simulink model "PubIfDecisionTOS_MDL"  (R2020b)
settings: configuration reference "DspaceConfig" (kept outside this file)
PostLoadFcn:
  | if any(exist('dsrtsu_mdlpostloadfcn', 'file') ~= 0), dsrtsu_mdlpostloadfcn('Execute', bdroot); end
InitFcn:
  | , if any(exist('dsmpb_private', 'file') ~= 0), dsmpb_private('dsmpb_mdlclblib', 'Init', bdroot); end,
undefined symbols (not defined in the file or in its folder): C_TOS_ACCEgoRAxletoFbumplength_m, C_TOS_ACCTargetFront_Flag, C_TOS_AEBJAPedObjDxThre_Val, C_TOS_AEBJAPedObjDyThre_Val, C_TOS_AEBJATargetSize_Val, C_TOS_AEBJAVehObjDxThre_Val, C_TOS_AEBJAVehObjDyThre_Val, C_TOS_AEBJuncPedTargetSize_Val, C_TOS_AEBLatObjDxThre_Val, C_TOS_AEBLatPedDyThre_Val, C_TOS_AEBLatTargetSize_Val, C_TOS_AEBLongTargetInEgoFront_Flag, C_TOS_axAbsGround_Parameter, C_TOS_CameraConfirmedFlag, C_TOS_CNsubjWidth, C_TOS_CurrentLaneCoreMinWidth_Val, C_TOS_CutInProb_Val_Zero, C_TOS_CutOutProb_Val_Zero, C_TOS_D2R_Val, C_TOS_DefaultValueObjectToCenterLine_dy, C_TOS_EgoCarWidth_Val, C_TOS_EgoDxRefPoint_m, C_TOS_EgoRAxletoFbumplength_m, C_TOS_HalfWidthVehicle_Con, C_TOS_HWA_CurrentLaneFlag, C_TOS_HWA_LeftLaneFlag, C_TOS_HWA_MovingDir_Vaild, C_TOS_HWA_MovState_Vaild, C_TOS_HWA_RightLaneFlag, C_TOS_LaneLineCourseErrorFront, C_TOS_LaneLineCourseErrorRear, C_TOS_MotorbikeDefaultWidth_m, C_TOS_NumberOfEffectiveTargets, C_TOS_Obj_Age_Val, C_TOS_Objdx_Constraint_Val, C_TOS_ObjectDefaultWidth_m, C_TOS_ObjInCurrentLane_Val, C_TOS_ObjInCurrentLaneValid, C_TOS_ObjInLeftLaneValid, C_TOS_ObjInRightLaneValid, C_TOS_ObjNotInCurrentLane_Val, C_TOS_ObjNotREElementType, C_TOS_ObjPredictDis_dy_ConstantVal_Zeros, C_TOS_ObjToCenterLine_ConstantVal_Zeros, C_TOS_OFMObjIDInvilad_Val, C_TOS_PIL_LatDisCons_Val_zero, C_TOS_PIL_ObjectCutInFlag_b, C_TOS_PIL_ObjectCutOutFlag_b, C_TOS_PIL_ObjLaneProb_al_Val, C_TOS_PP_ObjFusType_FC_Confirm_b, C_TOS_PP_ObjFusType_FC_FR_Confirm_b, C_TOS_PP_ObjFusType_FR_Confirm_b, C_TOS_RE_80BoolDefault_Val, C_TOS_RE_80Single181Default_Val, C_TOS_RE_80Single255Default_Val, C_TOS_RE_80Uint8Default_Val, C_TOS_RE_D2R, C_TOS_RE_D_180_Val, C_TOS_RE_InvalidObjectID_Val, C_TOS_RE_InvalidTargetChainDir_Val ... (+142)
libraries: simulink x1650, TOS_LIB x361, canfdmsglib x14
(part 11 of 69)

== system PubIfDecisionTOS_MDL/TOS_20201112/TOS_2012080320/PP1128/ISV_InputSignalVerification/LM_SignalVerif/LM_RR_Bus ==
  LM_LINE_RR : Inport
  Bus Creator2 : BusCreator  Inputs=8  OutDataTypeStr=Bus: TOS_LM_RR_Line_bus  NonVirtualBus=on
      settings: InheritFromInputs=off
  Bus Selector1 : BusSelector  OutputSignals=LM_Line01,LM_Line02,LM_Line03,LM_Line04,LM_Line05,LM_Line06,LM_Line07,LM_Line08
  LM_RR_Line01 : Subsystem
  LM_RR_Line02 : Subsystem
  LM_RR_Line03 : Subsystem
  LM_RR_Line04 : Subsystem
  LM_RR_Line05 : Subsystem
  LM_RR_Line06 : Subsystem
  LM_RR_Line07 : Subsystem
  LM_RR_Line08 : Subsystem
  LM_RR_Bus : Outport
  wires:
  LM_LINE_RR/1 -> Bus Selector1/1
  LM_RR_Line03/1(LM_RR_Line03) -> Bus Creator2/3  "LM_RR_Line03"
  LM_RR_Line02/1(LM_RR_Line02) -> Bus Creator2/2  "LM_RR_Line02"
  Bus Selector1/8 -> LM_RR_Line08/1(LM_Line08)  "<LM_Line08>"
  LM_RR_Line06/1(LM_RR_Line06) -> Bus Creator2/6  "LM_RR_Line06"
  LM_RR_Line04/1(LM_RR_Line04) -> Bus Creator2/4  "LM_RR_Line04"
  LM_RR_Line08/1(LM_RR_Line08) -> Bus Creator2/8  "LM_RR_Line08"
  Bus Selector1/2 -> LM_RR_Line02/1(LM_Line02)  "<LM_Line02>"
  Bus Selector1/6 -> LM_RR_Line06/1(LM_Line06)  "<LM_Line06>"
  LM_RR_Line05/1(LM_RR_Line05) -> Bus Creator2/5  "LM_RR_Line05"
  Bus Selector1/3 -> LM_RR_Line03/1(LM_Line03)  "<LM_Line03>"
  Bus Selector1/7 -> LM_RR_Line07/1(LM_Line07)  "<LM_Line07>"
  Bus Creator2/1 -> LM_RR_Bus/1
  LM_RR_Line01/1(LM_RR_Line01) -> Bus Creator2/1  "LM_RR_Line01"
  Bus Selector1/4 -> LM_RR_Line04/1(LM_Line04)  "<LM_Line04>"
  Bus Selector1/5 -> LM_RR_Line05/1(LM_Line05)  "<LM_Line05>"
  Bus Selector1/1 -> LM_RR_Line01/1(LM_Line01)  "<LM_Line01>"
  LM_RR_Line07/1(LM_RR_Line07) -> Bus Creator2/7  "LM_RR_Line07"

== system PubIfDecisionTOS_MDL/TOS_20201112/TOS_2012080320/TLJ/Pro/Pro/ObjInLane ==
  Object_Type : Inport
  Object_DY : Inport  Port=2
  PIL_CutinFlag : Inport  Port=3
  PIL_CutoutFlag : Inport  Port=4
  "PIL_EgoVehicleInLeftlaneProb  " : Inport  Port=5
  "PIL_EgoVehicleInMiddlelaneProb  " : Inport  Port=6
  "PIL_EgoVehicleInRightlaneProb  " : Inport  Port=7
  "PIL_ObjinLeftLaneProb " : Inport  Port=8
  PIL_ObjinEgoLaneProb : Inport  Port=9
  "PIL_ObjInRightlaneProb " : Inport  Port=10
  "TLJ_ObjinLeftLaneProb " : Inport  Port=11
  TLJ_ObjinEgoLaneProb : Inport  Port=12
  "TLJ_ObjInRightlaneProb " : Inport  Port=13
  Bus Creator1 : BusCreator  Inputs=13
  Bus Selector : BusSelector  OutputSignals=ObjInLeftLane_flag,ObjInEgoLane_flag,ObjInRightLane_flag,TOS_TLJ_ObjInLaneCondition_Flag_ObserVale
  Bus Selector1 : BusSelector  OutputSignals=Object_Type,TLJ_ObjinEgoLaneProb,TLJ_ObjinLeftLaneProb,TLJ_ObjInRightlaneProb,PIL_CutinFlag,PIL_CutoutFlag,Object_DY
  Bus Selector2 : BusSelector  OutputSignals=TLJ_ObjinEgoLaneProb,TLJ_ObjinLeftLaneProb,TLJ_ObjInRightlaneProb
  Bus Selector3 : BusSelector  OutputSignals=TLJ_ObjinEgoLaneProb,TLJ_ObjinLeftLaneProb,TLJ_ObjInRightlaneProb
  Bus Selector4 : BusSelector  OutputSignals=PIL_ObjinEgoLaneProb,PIL_ObjinLeftLaneProb,PIL_EgoVehicleInLeftlaneProb,PIL_EgoVehicleInMiddlelaneProb
  Bus Selector5 : BusSelector  OutputSignals=PIL_ObjinEgoLaneProb,PIL_ObjInRightlaneProb,PIL_EgoVehicleInRightlaneProb,PIL_EgoVehicleInMiddlelaneProb
  ObjInEgoLane_flag_1 : Subsystem  TreatAsAtomicUnit=on
  ObjInEgoLane_flag_2 : Subsystem  TreatAsAtomicUnit=on
  ObjInEgoLane_flag_3 : Subsystem  TreatAsAtomicUnit=on
  ObjInLane_Default : Subsystem  TreatAsAtomicUnit=on
  ObjInLeftLane_flag : Subsystem  TreatAsAtomicUnit=on
  ObjInRightLane_flag : Subsystem  TreatAsAtomicUnit=on
  Switch{,1..4} (5 alike) : Switch  Criteria=u2 > Threshold
  TLJ_ObjInEgoLane_1 : Subsystem
  TLJ_ObjInEgoLane_2 : Subsystem
  TLJ_ObjInEgoLane_3 : Subsystem
  TLJ_ObjInLeftLane : Subsystem
  TLJ_ObjInRightLane : Subsystem
  TLJ_ObjInLeftLane_flag : Outport
  TLJ_ObjInEgoLane_flag : Outport  Port=2
  TLJ_ObjInRightLane_flag : Outport  Port=3
  TOS_TLJ_ObjInLaneCondition_Flag_ObserVale : Outport  Port=4
  wires:
  ObjInLane_Default/1(ObjInEgoLane_flag_2) -> Switch4/3
  ObjInEgoLane_flag_1/1(ObjInEgoLane_flag_1) -> Switch/1
  Bus Selector5/3 -> TLJ_ObjInEgoLane_3/3("PIL_EgoVehicleInRightlaneProb  ")  "<PIL_EgoVehicleInRightlaneProb>"
  TLJ_ObjInEgoLane_3/1(TLJ_ObjInRightLane_flag) -> Switch4/2  "TLJ_ObjInEgoLane_3"
  Bus Selector2/1 -> TLJ_ObjInLeftLane/1(TLJ_ObjinEgoLaneProb)  "<TLJ_ObjinEgoLaneProb>"
  "PIL_EgoVehicleInLeftlaneProb  "/1 -> Bus Creator1/5  "PIL_EgoVehicleInLeftlaneProb"
  Bus Selector3/2 -> TLJ_ObjInRightLane/2(TLJ_ObjinLeftLaneProb)  "<TLJ_ObjinLeftLaneProb>"
  PIL_CutinFlag/1 -> Bus Creator1/3  "PIL_CutinFlag"
  Bus Selector3/3 -> TLJ_ObjInRightLane/3(TLJ_ObjinRightLaneProb)  "<TLJ_ObjInRightlaneProb>"
  Switch4/1 -> Switch3/3
  TLJ_ObjInLeftLane/1(TLJ_ObjInLeftLane_flag) -> Switch1/2  "TLJ_ObjInLeftLane"
  Switch/1 -> Bus Selector/1
  TLJ_ObjInEgoLane_2/1(TLJ_ObjInRightLane_flag) -> Switch3/2  "TLJ_ObjInEgoLane_2"
  TLJ_ObjInRightLane/1(TLJ_ObjInRightLane_flag) -> Switch2/2  "TLJ_ObjInRightLane"
  ObjInEgoLane_flag_3/1(ObjInEgoLane_flag_1) -> Switch4/1
  TLJ_ObjInEgoLane_1/1(TLJ_ObjInEgoLane_flag) -> Switch/2  "TLJ_ObjInEgoLane_1"
  ObjInRightLane_flag/1(ObjInRightLane_flag) -> Switch2/1
  Bus Selector1/4 -> TLJ_ObjInEgoLane_1/4("TLJ_ObjInRightlaneProb ")  "<TLJ_ObjInRightlaneProb>"
  ObjInEgoLane_flag_2/1(ObjInEgoLane_flag_1) -> Switch3/1
  Bus Selector5/1 -> TLJ_ObjInEgoLane_3/1("PIL_ObjinEgoLaneProb ")  "<PIL_ObjinEgoLaneProb>"
  Bus Creator1/1 -> Bus Selector5/1, Bus Selector4/1, Bus Selector3/1, Bus Selector2/1, Bus Selector1/1
  Bus Selector1/1 -> TLJ_ObjInEgoLane_1/1(Object_Type)  "<Object_Type>"
  Object_Type/1 -> Bus Creator1/1  "Object_Type"
  "PIL_EgoVehicleInMiddlelaneProb  "/1 -> Bus Creator1/6  "PIL_EgoVehicleInMiddlelaneProb"
  TLJ_ObjinEgoLaneProb/1 -> Bus Creator1/12  "TLJ_ObjinEgoLaneProb"
  Bus Selector4/3 -> TLJ_ObjInEgoLane_2/3("PIL_EgoVehicleInLeftlaneProb  ")  "<PIL_EgoVehicleInLeftlaneProb>"
  "PIL_EgoVehicleInRightlaneProb  "/1 -> Bus Creator1/7  "PIL_EgoVehicleInRightlaneProb"
  Bus Selector1/5 -> TLJ_ObjInEgoLane_1/5(PIL_CutinFlag)  "<PIL_CutinFlag>"
  "TLJ_ObjInRightlaneProb "/1 -> Bus Creator1/13  "TLJ_ObjInRightlaneProb"
  Bus Selector2/3 -> TLJ_ObjInLeftLane/3(TLJ_ObjinRightLaneProb)  "<TLJ_ObjInRightlaneProb>"
  "TLJ_ObjinLeftLaneProb "/1 -> Bus Creator1/11  "TLJ_ObjinLeftLaneProb"
  Bus Selector4/1 -> TLJ_ObjInEgoLane_2/1("PIL_ObjinEgoLaneProb ")  "<PIL_ObjinEgoLaneProb>"
  Switch3/1 -> Switch2/3
  Bus Selector2/2 -> TLJ_ObjInLeftLane/2("TLJ_ObjinLeftLaneProb ")  "<TLJ_ObjinLeftLaneProb>"
  ObjInLeftLane_flag/1(ObjInLeftLane_flag) -> Switch1/1
  Bus Selector3/1 -> TLJ_ObjInRightLane/1(TLJ_ObjinEgoLaneProb)  "<TLJ_ObjinEgoLaneProb>"
  Bus Selector4/4 -> TLJ_ObjInEgoLane_2/4("PIL_EgoVehicleInMiddlelaneProb  ")  "<PIL_EgoVehicleInMiddlelaneProb>"
  Switch1/1 -> Switch/3
  Bus Selector4/2 -> TLJ_ObjInEgoLane_2/2("PIL_ObjInLeftlaneProb ")  "<PIL_ObjinLeftLaneProb>"
  Switch2/1 -> Switch1/3
  Bus Selector1/2 -> TLJ_ObjInEgoLane_1/2(TLJ_ObjinEgoLaneProb)  "<TLJ_ObjinEgoLaneProb>"
  Bus Selector5/2 -> TLJ_ObjInEgoLane_3/2("PIL_ObjInRightlaneProb ")  "<PIL_ObjInRightlaneProb>"
  Bus Selector1/3 -> TLJ_ObjInEgoLane_1/3("TLJ_ObjinLeftLaneProb ")  "<TLJ_ObjinLeftLaneProb>"
  Bus Selector5/4 -> TLJ_ObjInEgoLane_3/4("PIL_EgoVehicleInMiddlelaneProb  ")  "<PIL_EgoVehicleInMiddlelaneProb>"
  Bus Selector/1 -> TLJ_ObjInLeftLane_flag/1  "<ObjInLeftLane_flag>"
  Bus Selector/2 -> TLJ_ObjInEgoLane_flag/1  "<ObjInEgoLane_flag>"
  Bus Selector/3 -> TLJ_ObjInRightLane_flag/1  "<ObjInRightLane_flag>"
  "PIL_ObjinLeftLaneProb "/1 -> Bus Creator1/8  "PIL_ObjinLeftLaneProb"
  PIL_ObjinEgoLaneProb/1 -> Bus Creator1/9  "PIL_ObjinEgoLaneProb"
  "PIL_ObjInRightlaneProb "/1 -> Bus Creator1/10  "PIL_ObjInRightlaneProb"
  Bus Selector/4 -> TOS_TLJ_ObjInLaneCondition_Flag_ObserVale/1  "<TOS_TLJ_ObjInLaneCondition_Flag_ObserVale>"
  Object_DY/1 -> Bus Creator1/2  "Object_DY"
  Bus Selector1/7 -> TLJ_ObjInEgoLane_1/7(Object_DY)  "<Object_DY>"
  PIL_CutoutFlag/1 -> Bus Creator1/4  "PIL_CutoutFlag"
  Bus Selector1/6 -> TLJ_ObjInEgoLane_1/6(PIL_CutoutFlag)  "<PIL_CutoutFlag>"

== system PubIfDecisionTOS_MDL/TOS_20201112/TOS_2012080320/TLJ/Pro/Pro/Pro ==
  PIL_EgoLaneProb : Inport
  PIL_LeftLaneProb : Inport  Port=2
  PIL_RightLaneProb : Inport  Port=3
  PIL_EgoVehicle_EgoLaneProb : Inport  Port=4
  PIL_EgoVehicle_LeftLaneProb : Inport  Port=5
  PIL_EgoVehicle_RightLaneProb : Inport  Port=6
  Add1 : Sum  OutDataTypeStr=single
  Add2 : Sum  OutDataTypeStr=single
  Add3 : Sum  Inputs=+++  OutDataTypeStr=single
  Bus Creator : BusCreator  Inputs=6
  Bus Selector : BusSelector  OutputSignals=ObjLaneProb_ix_i0,EgoLaneProb_i0,ObjLaneProb_ix_i1,EgoLaneProb_i1,ObjLaneProb_ix_i2,EgoLaneProb_i2
  Bus Selector1 : BusSelector  OutputSignals=ObjLaneProb_ix_i0,EgoLaneProb_i1,ObjLaneProb_ix_i1,EgoLaneProb_i2
  Bus Selector2 : BusSelector  OutputSignals=ObjLaneProb_ix_i1,EgoLaneProb_i0,ObjLaneProb_ix_i2,EgoLaneProb_i1
  Product{1..7} (7 alike) : Product
  TLJ_ObjinLeftLaneProb : Outport
  TLJ_ObjinEgoLaneProb : Outport  Port=2
  TLJ_ObjinRightLaneProb : Outport  Port=3
  wires:
  Add1/1 -> TLJ_ObjinLeftLaneProb/1
  Bus Selector1/2 -> Product3/2  "<EgoLaneProb_i1>"
  Bus Selector/1 -> Product1/1  "<ObjLaneProb_ix_i0>"
  Bus Selector1/3 -> Product4/1  "<ObjLaneProb_ix_i1>"
  PIL_LeftLaneProb/1 -> Bus Creator/1  "ObjLaneProb_ix_i0"
  Bus Selector/6 -> Product7/2  "<EgoLaneProb_i2>"
  Bus Selector/2 -> Product1/2  "<EgoLaneProb_i0>"
  Product7/1 -> Add3/3
  Product1/1 -> Add3/1
  Bus Selector1/1 -> Product3/1  "<ObjLaneProb_ix_i0>"
  PIL_EgoVehicle_EgoLaneProb/1 -> Bus Creator/5  "EgoLaneProb_i1"
  Bus Selector/5 -> Product7/1  "<ObjLaneProb_ix_i2>"
  Bus Creator/1 -> Bus Selector2/1, Bus Selector1/1, Bus Selector/1
  PIL_EgoVehicle_RightLaneProb/1 -> Bus Creator/6  "EgoLaneProb_i2"
  Bus Selector/4 -> Product2/2  "<EgoLaneProb_i1>"
  Add3/1 -> TLJ_ObjinEgoLaneProb/1
  PIL_EgoVehicle_LeftLaneProb/1 -> Bus Creator/4  "EgoLaneProb_i0"
  Product6/1 -> Add2/2
  Bus Selector/3 -> Product2/1  "<ObjLaneProb_ix_i1>"
  PIL_RightLaneProb/1 -> Bus Creator/3  "ObjLaneProb_ix_i2"
  Bus Selector2/1 -> Product5/1  "<ObjLaneProb_ix_i1>"
  Product4/1 -> Add1/2
  Product2/1 -> Add3/2
  Bus Selector1/4 -> Product4/2  "<EgoLaneProb_i2>"
  PIL_EgoLaneProb/1 -> Bus Creator/2  "ObjLaneProb_ix_i1"
  Bus Selector2/3 -> Product6/1  "<ObjLaneProb_ix_i2>"
  Product3/1 -> Add1/1
  Product5/1 -> Add2/1
  Bus Selector2/2 -> Product5/2  "<EgoLaneProb_i0>"
  Add2/1 -> TLJ_ObjinRightLaneProb/1
  Bus Selector2/4 -> Product6/2  "<EgoLaneProb_i1>"

== system PubIfDecisionTOS_MDL/TOS_20201112/TOS_2012080320/TOS/ACC/TOS_ACCCurrentLane/ACCTargetInfor ==
  note: TOS_ProbInLaneCalculat 信号未使用
  OFM_SignalVerification : Inport
  TOS_AddAttributes : Inport  Port=2
  TOS_ProbInLaneCalculat : Inport  Port=3
  TOS_ACCP0TargetIndex : Inport  Port=4  OutDataTypeStr=uint8
  TOS_ACCP1TargetIndex : Inport  Port=5  OutDataTypeStr=uint8
  Bus Creator : BusCreator  Inputs=3
  Bus Selector : BusSelector  OutputSignals=OFM_SignalVerification,TOS_AddAttributes,TOS_ProbInLaneCalculat
  Bus Selector1 : BusSelector  OutputSignals=OFM_SignalVerification,TOS_AddAttributes
  Bus Selector2 : BusSelector  OutputSignals=IDP0
  TOS_ACCP0TargetInfor : Stateflow chart  TreatAsAtomicUnit=on
  TOS_ACCP1TargetInfor : Stateflow chart  TreatAsAtomicUnit=on
  TOS_ACCP0 : Outport  PortDimensions=1  BusOutputAsStruct=on
  TOS_ACCP1 : Outport  Port=2
  wires:
  TOS_ACCP1TargetInfor/1(TOS_ACCPO1TargetInfo) -> TOS_ACCP1/1
  Bus Selector1/2 -> TOS_ACCP1TargetInfor/3(TOS_AddAttributes)  "<TOS_AddAttributes>"
  Bus Selector1/1 -> TOS_ACCP1TargetInfor/2(OFM_SignalVerification)  "<OFM_SignalVerification>"
  TOS_ACCP0TargetInfor/1(TOS_ACCPO0TargetInfo) -> Bus Selector2/1, TOS_ACCP0/1
  Bus Selector/3 -> TOS_ACCP0TargetInfor/3(TOS_ProbInLaneCalculat)  "<TOS_ProbInLaneCalculat>"
  TOS_ProbInLaneCalculat/1 -> Bus Creator/3  "TOS_ProbInLaneCalculat"
  OFM_SignalVerification/1 -> Bus Creator/1  "OFM_SignalVerification"
  TOS_AddAttributes/1 -> Bus Creator/2  "TOS_AddAttributes"
  Bus Selector/2 -> TOS_ACCP0TargetInfor/2(TOS_AddAttributes)  "<TOS_AddAttributes>"
  Bus Selector/1 -> TOS_ACCP0TargetInfor/1(OFM_SignalVerification)  "<OFM_SignalVerification>"
  Bus Selector2/1 -> [TOS_ACCP0_ID]  "<IDP0>"
  TOS_ACCP0TargetIndex/1 -> TOS_ACCP0TargetInfor/4(TOS_ACCPO0TargetIndex)
  TOS_ACCP1TargetIndex/1 -> TOS_ACCP1TargetInfor/4(TOS_ACCPO1TargetIndex)
  [TOS_ACCP0_ID] -> TOS_ACCP1TargetInfor/1(IDP0)
  Bus Creator/1 -> Bus Selector1/1, Bus Selector/1

== system PubIfDecisionTOS_MDL/TOS_20201112/TOS_2012080320/TOS/ACC/TOS_ACCCurrentLane/ACC_CurrentLane_Target ==
  VIE_EgoVelocity : Inport
  OFM_SignalVerification : Inport  Port=2
  TOS_AddAttributes : Inport  Port=3
  TOS_TLJ_SameLaneConfirm_Flag : Inport  Port=4
  TOS_ProbInLaneCalculat : Inport  Port=5
  TOS_VCAN_SignalVerification : Inport  Port=6
  LM_LR_Line04_dDisStart : Inport  Port=7
  LM_LR_Line04_dDisEnd : Inport  Port=8
  LM_LR_Line05_dDisStart : Inport  Port=9
  LM_LR_Line05_dDisEnd : Inport  Port=10
  LM_LR_Line06_dDisStart : Inport  Port=11
  LM_LR_Line06_dDisEnd : Inport  Port=12
  LM_LR_Line04_pC2 : Inport  Port=13
  LM_LR_Line05_pC2 : Inport  Port=14
  LM_LR_Line06_pC2 : Inport  Port=15
  LM_LR_Line04_fCamValid : Inport  Port=16
  LM_LR_Line05_fCamValid : Inport  Port=17
  LM_LR_Line06_fCamValid : Inport  Port=18
  LM_LR_Line04_pC0 : Inport  Port=19
  LM_RL_Line04_pC0 : Inport  Port=20
  LM_LR_Line04_pC1 : Inport  Port=21
  LM_RL_Line04_pC1 : Inport  Port=22
  ACC_P0_P1_Index : Inport  Port=23
  ACC_TargetP0_ID_K1 : Inport  Port=24
  ACC_TargetP0_MovState_K1 : Inport  Port=25
  ACC_TargetP1_ID_K1 : Inport  Port=26
  ACC_TargetP1_MovState_K1 : Inport  Port=27
  ACC_TargetP0_ID_K2 : InportShadow  Port=24
  ACC_TargetP0_MovState_K2 : InportShadow  Port=25
  ACC_TargetP1_ID_K2 : InportShadow  Port=26
  ACC_TargetP1_MovState_K2 : InportShadow  Port=27
  Bus Creator : BusCreator  Inputs=31
  Bus Creator1 : BusCreator  Inputs=18
  Bus Creator2 : BusCreator  Inputs=18
  Bus Selector : BusSelector  OutputSignals=ACC_P0_P1_Index,OFM_SignalVerification.Object_ID,OFM_SignalVerification.Object_Fus_Type,OFM_SignalVerification.Object_MovingState,TOS_AddAttributes.PP_ObjMovingDirSignalProcessing,OFM_SignalVerification.Object_HeadingAngle,OFM_SignalVerification.Object_DX,TOS_TLJ_SameLaneConfirm_Flag,OFM_SignalVerification.Object_Type,OFM_SignalVerification.Object_ObstacleProb,OFM_SignalVerification.Object_DY,TOS_AddAttributes.PP_ObjFusType_FC_FR_Confirm,TOS_AddAttributes.PP_ObjFusType_FR_Confirm,TOS_AddAttributes.PP_ObjFusType_FC_Confirm,OFM_SignalVerification.Object_VX,OFM_SignalVerification.Object_VY,VIE_EgoVelocity,TOS_VCAN_SignalVerification.SteerWheelAng,TOS_ProbInLaneCalculat.PIL_OverlapRatio,ACC_TargetP0_ID_K1,ACC_TargetP0_ID_K2,ACC_TargetP0_MovState_K1,ACC_TargetP0_MovState_K2,LM_LR_Line04_dDisStart,LM_LR_Line04_dDisEnd,LM_LR_Line05_dDisStart,LM_LR_Line05_dDisEnd,LM_LR_Line06_dDisStart,LM_LR_Line06_dDisEnd,LM_LR_Line04_pC2,LM_LR_Line05_pC2,LM_LR_Line06_pC2,LM_LR_Line04_fCamValid,LM_LR_Line05_fCamValid,LM_LR_Line06_fCamValid,LM_LR_Line04_pC0,LM_RL_Line04_pC0,LM_LR_Line04_pC1,LM_RL_Line04_pC1
  Bus Selector2 : BusSelector  OutputSignals=ACC_P0_P1_Index,OFM_SignalVerification.Object_ID,OFM_SignalVerification.Object_Fus_Type,OFM_SignalVerification.Object_MovingState,TOS_AddAttributes.PP_ObjMovingDirSignalProcessing,OFM_SignalVerification.Object_HeadingAngle,OFM_SignalVerification.Object_DX,TOS_TLJ_SameLaneConfirm_Flag,OFM_SignalVerification.Object_Type,OFM_SignalVerification.Object_ObstacleProb,OFM_SignalVerification.Object_DY,TOS_AddAttributes.PP_ObjFusType_FC_FR_Confirm,TOS_AddAttributes.PP_ObjFusType_FR_Confirm,TOS_AddAttributes.PP_ObjFusType_FC_Confirm,OFM_SignalVerification.Object_VX,OFM_SignalVerification.Object_VY,VIE_EgoVelocity,TOS_VCAN_SignalVerification.SteerWheelAng,TOS_ProbInLaneCalculat.PIL_OverlapRatio,ACC_TargetP1_ID_K1,ACC_TargetP1_ID_K2,ACC_TargetP1_MovState_K1,ACC_TargetP1_MovState_K2,LM_LR_Line04_dDisStart,LM_LR_Line04_dDisEnd,LM_LR_Line05_dDisStart,LM_LR_Line05_dDisEnd,LM_LR_Line06_dDisStart,LM_LR_Line06_dDisEnd,LM_LR_Line04_pC2,LM_LR_Line05_pC2,LM_LR_Line06_pC2,LM_LR_Line04_fCamValid,LM_LR_Line05_fCamValid,LM_LR_Line06_fCamValid,LM_LR_Line04_pC0,LM_RL_Line04_pC0
  Data Type Conversion{1..4} (4 alike) : DataTypeConversion  OutDataTypeStr=Enum: ObjectMovingState_E
  Delay{,3..4,7} (4 alike) : Delay  InitialCondition=0
  Delay{1..2,5..6} (4 alike) : Delay  DelayLength=1  InitialCondition=0
  TOS_ACC_P0 : Subsystem
  TOS_ACC_P1 : Subsystem
  Terminator : Terminator
  Terminator1 : Terminator
  TOS_ACC_P0_TragetIndex : Outport
  TOS_ACC_P1_TragetIndex : Outport  Port=2
  wires:
  TOS_TLJ_SameLaneConfirm_Flag/1 -> Bus Creator/4  "TOS_TLJ_SameLaneConfirm_Flag"
  TOS_AddAttributes/1 -> Bus Creator/3  "TOS_AddAttributes"
  OFM_SignalVerification/1 -> Bus Creator/2  "OFM_SignalVerification"
  VIE_EgoVelocity/1 -> Bus Creator/1  "VIE_EgoVelocity"
  TOS_ProbInLaneCalculat/1 -> Bus Creator/5  "TOS_ProbInLaneCalculat"
  Bus Selector/3 -> TOS_ACC_P0/3(Object_Fus_Type)  "<Object_Fus_Type>"
  Bus Selector/4 -> TOS_ACC_P0/4(object_MovingState)  "<Object_MovingState>"
  TOS_ACC_P0/1(TOS_ACC_P0_Index) -> [TOS_ACC_P0_TragetIndex], TOS_ACC_P0_TragetIndex/1  "TOS_ACC_P0_TragetIndex"
  Bus Selector/7 -> TOS_ACC_P0/7(Object_DX)  "<Object_DX>"
  Bus Selector/8 -> TOS_ACC_P0/8(TOS_TLJ_SameLaneConfirm_Flag)  "<TOS_TLJ_SameLaneConfirm_Flag>"
  Bus Selector/9 -> TOS_ACC_P0/9(Object_Type)  "<Object_Type>"
  Bus Selector/2 -> TOS_ACC_P0/2(Object_ID)  "<Object_ID>"
  TOS_ACC_P0/2(TOS_ACC_FusionType_ObserVale) -> Bus Creator1/1  "TOS_ACC_P0_FusionType_ObserVale"
  TOS_ACC_P0/3(TOS_ACC_TrgMovDir_ObserVale) -> Bus Creator1/2  "TOS_ACC_P0_TrgMovDir_ObserVale"
  TOS_ACC_P0/4(TOS_ACC_TargetDxConfirm_ObserVale) -> Bus Creator1/3  "TOS_ACC_P0_TargetDxConfirm_ObserVale"
  TOS_ACC_P0/5(TOS_ACC_ObjType_ObserVale) -> Bus Creator1/4  "TOS_ACC_P0_ObjType_ObserVale"
  Bus Selector/10 -> TOS_ACC_P0/10(Object_ObstacleProb)  "<Object_ObstacleProb>"
  TOS_ACC_P0/6(TOS_ACC_ObstacleProb_ObserVale) -> Bus Creator1/5  "TOS_ACC_P0_ObstacleProb_ObserVale"
  Bus Selector/5 -> TOS_ACC_P0/5(PP_ObjMovingDirSignalProcessing)  "<PP_ObjMovingDirSignalProcessing>"
  Bus Selector/6 -> TOS_ACC_P0/6(Object_HeadingAngle)  "<Object_HeadingAngle>"
  Bus Selector/11 -> TOS_ACC_P0/11(Object_DY)  "<Object_DY>"
  TOS_ACC_P0/7(TOS_ACC_DyConfirm_ObserVale) -> Bus Creator1/6  "TOS_ACC_P0_DyConfirm_ObserVale"
  Bus Creator1/1 -> [TOS_ACC_P0_ObserVale], Terminator/1  "TOS_ACC_P0_ObserVale"
  ACC_P0_P1_Index/1 -> Bus Creator/23  "ACC_P0_P1_Index"
  Bus Selector/1 -> TOS_ACC_P0/1(ACC_P0_P1_Index)  "<ACC_P0_P1_Index>"
  Bus Selector/12 -> TOS_ACC_P0/12(PP_ObjFusType_FC_FR_Confirm)  "<PP_ObjFusType_FC_FR_Confirm>"
  Bus Selector/13 -> TOS_ACC_P0/13(PP_ObjFusType_FR_Confirm)  "<PP_ObjFusType_FR_Confirm>"
  Bus Selector/14 -> TOS_ACC_P0/14(PP_ObjFusType_FC_Confirm)  "<PP_ObjFusType_FC_Confirm>"
  Bus Selector/15 -> TOS_ACC_P0/15(Object_VX)  "<Object_VX>"
  Bus Selector/16 -> TOS_ACC_P0/16(Object_VY)  "<Object_VY>"
  Bus Selector/17 -> TOS_ACC_P0/17(VIE_EgoVelocity)  "<VIE_EgoVelocity>"
  TOS_VCAN_SignalVerification/1 -> Bus Creator/6  "TOS_VCAN_SignalVerification"
  Bus Selector/18 -> TOS_ACC_P0/18(SteerWheelAng)  "<SteerWheelAng>"
  Bus Selector/19 -> TOS_ACC_P0/19(PIL_OverlapRatio)  "<PIL_OverlapRatio>"
  TOS_ACC_P0/17(TOS_ACC_DyConfirm_4_OverlapRatio_ObserVale) -> Bus Creator1/16  "TOS_ACC_P0_DyConfirm_4_OverlapRatio_ObserVale"
  Delay1/1 -> Bus Creator/24  "ACC_TargetP0_ID_K1"
  Delay/1 -> Bus Creator/25  "ACC_TargetP0_ID_K2"
  Delay2/1 -> Data Type Conversion2/1
  Data Type Conversion1/1 -> Bus Creator/27  "ACC_TargetP0_MovState_K2"
  Bus Selector/20 -> TOS_ACC_P0/20(ACC_TargetP0_ID_K1)  "<ACC_TargetP0_ID_K1>"
  Bus Selector/21 -> TOS_ACC_P0/21(ACC_TargetP0_ID_K2)  "<ACC_TargetP0_ID_K2>"
  Bus Selector/22 -> TOS_ACC_P0/22(ACC_TargetP0_MovState_K1)  "<ACC_TargetP0_MovState_K1>"
  Bus Selector/23 -> TOS_ACC_P0/23(ACC_TargetP0_MovState_K2)  "<ACC_TargetP0_MovState_K2>"
  ACC_TargetP0_MovState_K2/1 -> Delay3/1
  Data Type Conversion2/1 -> Bus Creator/26  "ACC_TargetP0_MovState_K1"
  Bus Creator/1 -> Bus Selector2/1, Bus Selector/1
  TOS_ACC_P0/8(TOS_ACC_TrgMovDirFlag_1_ObserVale) -> Bus Creator1/7  "TOS_ACC_P0_TrgMovDirFlag_1_ObserVale"
  TOS_ACC_P0/9(TOS_ACC_TrgMovDirFlag_2_ObserVale) -> Bus Creator1/8  "TOS_ACC_P0_TrgMovDirFlag_2_ObserVale"
  TOS_ACC_P0/10(TOS_ACC_TrgMovDirFlag_3_ObserVale) -> Bus Creator1/9  "TOS_ACC_P0_TrgMovDirFlag_3_ObserVale"
  TOS_ACC_P0/11(TOS_ACC_TrgMovDirFlag_4_ObserVale) -> Bus Creator1/10  "TOS_ACC_P0_TrgMovDirFlag_4_ObserVale"
  TOS_ACC_P0/12(TOS_ACC_TrgMovDirFlag_5_ObserVale) -> Bus Creator1/11  "TOS_ACC_P0_TrgMovDirFlag_5_ObserVale"
  TOS_ACC_P0/14(TOS_ACC_DyConfirm_1_ObserVale) -> Bus Creator1/13  "TOS_ACC_P0_DyConfirm_1_ObserVale"
  TOS_ACC_P0/15(TOS_ACC_DyConfirm_2_ObserVale) -> Bus Creator1/14  "TOS_ACC_P0_DyConfirm_2_ObserVale"
  TOS_ACC_P0/16(TOS_ACC_DyConfirm_3_ObserVale) -> Bus Creator1/15  "TOS_ACC_P0_DyConfirm_3_ObserVale"
  TOS_ACC_P1/16(TOS_ACC_DyConfirm_3_ObserVale) -> Bus Creator2/15  "TOS_ACC_P1_DyConfirm_3_ObserVale"
  TOS_ACC_P1/15(TOS_ACC_DyConfirm_2_ObserVale) -> Bus Creator2/14  "TOS_ACC_P1_DyConfirm_2_ObserVale"
  TOS_ACC_P1/14(TOS_ACC_DyConfirm_1_ObserVale) -> Bus Creator2/13  "TOS_ACC_P1_DyConfirm_1_ObserVale"
  TOS_ACC_P1/12(TOS_ACC_TrgMovDirFlag_5_ObserVale) -> Bus Creator2/11  "TOS_ACC_P1_TrgMovDirFlag_5_ObserVale"
  TOS_ACC_P1/11(TOS_ACC_TrgMovDirFlag_4_ObserVale) -> Bus Creator2/10  "TOS_ACC_P1_TrgMovDirFlag_4_ObserVale"
  TOS_ACC_P1/10(TOS_ACC_TrgMovDirFlag_3_ObserVale) -> Bus Creator2/9  "TOS_ACC_P1_TrgMovDirFlag_3_ObserVale"
  TOS_ACC_P1/9(TOS_ACC_TrgMovDirFlag_2_ObserVale) -> Bus Creator2/8  "TOS_ACC_P1_TrgMovDirFlag_2_ObserVale"
  TOS_ACC_P1/8(TOS_ACC_TrgMovDirFlag_1_ObserVale) -> Bus Creator2/7  "TOS_ACC_P1_TrgMovDirFlag_1_ObserVale"
  Bus Creator2/1 -> [TOS_ACC_P1_ObserVale], Terminator1/1  "TOS_ACC_P1_ObserVale"
  TOS_ACC_P1/7(TOS_ACC_DyConfirm_ObserVale) -> Bus Creator2/6  "TOS_ACC_P1_DyConfirm_ObserVale"
  TOS_ACC_P1/6(TOS_ACC_ObstacleProb_ObserVale) -> Bus Creator2/5  "TOS_ACC_P1_ObstacleProb_ObserVale"
  TOS_ACC_P1/5(TOS_ACC_ObjType_ObserVale) -> Bus Creator2/4  "TOS_ACC_P1_ObjType_ObserVale"
  TOS_ACC_P1/4(TOS_ACC_TargetDxConfirm_ObserVale) -> Bus Creator2/3  "TOS_ACC_P1_TargetDxConfirm_ObserVale"
  TOS_ACC_P1/3(TOS_ACC_TrgMovDir_ObserVale) -> Bus Creator2/2  "TOS_ACC_P1_TrgMovDir_ObserVale"
  TOS_ACC_P1/2(TOS_ACC_FusionType_ObserVale) -> Bus Creator2/1  "TOS_ACC_P1_FusionType_ObserVale"
  TOS_ACC_P1/1(TOS_ACC_P1_Index) -> [TOS_ACC_P1_TragetIndex], TOS_ACC_P1_TragetIndex/1  "TOS_ACC_P1_TragetIndex"
  Delay3/1 -> Data Type Conversion1/1
  ACC_TargetP0_ID_K2/1 -> Delay/1
  ACC_TargetP0_ID_K1/1 -> Delay1/1
  ACC_TargetP0_MovState_K1/1 -> Delay2/1
  ACC_TargetP1_ID_K2/1 -> Delay4/1
  ACC_TargetP1_ID_K1/1 -> Delay5/1
  ACC_TargetP1_MovState_K1/1 -> Delay6/1
  ACC_TargetP1_MovState_K2/1 -> Delay7/1
  Delay5/1 -> Bus Creator/28  "ACC_TargetP1_ID_K1"
  Delay4/1 -> Bus Creator/29  "ACC_TargetP1_ID_K2"
  Delay6/1 -> Data Type Conversion4/1
  Delay7/1 -> Data Type Conversion3/1
  Data Type Conversion3/1 -> Bus Creator/31  "ACC_TargetP1_MovState_K2"
  Data Type Conversion4/1 -> Bus Creator/30  "ACC_TargetP1_MovState_K1"
  TOS_ACC_P0/13(TOS_ACC_TrgMovDirFlag_6_ObserVale) -> Bus Creator1/12  "TOS_ACC_P0_TrgMovDirFlag_6_ObserVale"
  LM_LR_Line04_dDisStart/1 -> Bus Creator/7  "LM_LR_Line04_dDisStart"
  LM_LR_Line04_dDisEnd/1 -> Bus Creator/8  "LM_LR_Line04_dDisEnd"
  LM_LR_Line05_dDisStart/1 -> Bus Creator/9  "LM_LR_Line05_dDisStart"
  LM_LR_Line05_dDisEnd/1 -> Bus Creator/10  "LM_LR_Line05_dDisEnd"
  LM_LR_Line06_dDisStart/1 -> Bus Creator/11  "LM_LR_Line06_dDisStart"
  LM_LR_Line06_dDisEnd/1 -> Bus Creator/12  "LM_LR_Line06_dDisEnd"
  LM_LR_Line04_pC2/1 -> Bus Creator/13  "LM_LR_Line04_pC2"
  LM_LR_Line05_pC2/1 -> Bus Creator/14  "LM_LR_Line05_pC2"
  LM_LR_Line06_pC2/1 -> Bus Creator/15  "LM_LR_Line06_pC2"
  Bus Selector/24 -> TOS_ACC_P0/24(LM_LR_Line04_dDisStart)  "<LM_LR_Line04_dDisStart>"
  Bus Selector/25 -> TOS_ACC_P0/25(LM_LR_Line04_dDisEnd)  "<LM_LR_Line04_dDisEnd>"
  Bus Selector/26 -> TOS_ACC_P0/26(LM_LR_Line05_dDisStart)  "<LM_LR_Line05_dDisStart>"
  Bus Selector/27 -> TOS_ACC_P0/27(LM_LR_Line05_dDisEnd)  "<LM_LR_Line05_dDisEnd>"
  Bus Selector/28 -> TOS_ACC_P0/28(LM_LR_Line06_dDisStart)  "<LM_LR_Line06_dDisStart>"
  Bus Selector/29 -> TOS_ACC_P0/29(LM_LR_Line06_dDisEnd)  "<LM_LR_Line06_dDisEnd>"
  Bus Selector/30 -> TOS_ACC_P0/30(LM_LR_Line04_pC2)  "<LM_LR_Line04_pC2>"
  Bus Selector/31 -> TOS_ACC_P0/31(LM_LR_Line05_pC2)  "<LM_LR_Line05_pC2>"
  Bus Selector/32 -> TOS_ACC_P0/32(LM_LR_Line06_pC2)  "<LM_LR_Line06_pC2>"
  LM_LR_Line04_fCamValid/1 -> Bus Creator/16  "LM_LR_Line04_fCamValid"
  LM_LR_Line05_fCamValid/1 -> Bus Creator/17  "LM_LR_Line05_fCamValid"
  LM_LR_Line06_fCamValid/1 -> Bus Creator/18  "LM_LR_Line06_fCamValid"
  Bus Selector/33 -> TOS_ACC_P0/33(LM_LR_Line04_fCamValid)  "<LM_LR_Line04_fCamValid>"
  Bus Selector/34 -> TOS_ACC_P0/34(LM_LR_Line05_fCamValid)  "<LM_LR_Line05_fCamValid>"
  Bus Selector/35 -> TOS_ACC_P0/35(LM_LR_Line06_fCamValid)  "<LM_LR_Line06_fCamValid>"
  TOS_ACC_P0/18(TOS_ACC_DyConfirm_5_OverlapConfirm_ObserVale) -> Bus Creator1/17  "TOS_ACC_P0_DyConfirm_5_OverlapConfirm_ObserVale"
  TOS_ACC_P0/19(TOS_ACC_DyConfirm_ALL_6_ObserVale) -> Bus Creator1/18  "TOS_ACC_P0_DyConfirm_ALL_6_ObserVale"
  LM_LR_Line04_pC0/1 -> Bus Creator/19  "LM_LR_Line04_pC0"
  LM_RL_Line04_pC0/1 -> Bus Creator/20  "LM_RL_Line04_pC0"
  Bus Selector/36 -> TOS_ACC_P0/36(LM_LR_Line04_pC0)  "<LM_LR_Line04_pC0>"
  Bus Selector/37 -> TOS_ACC_P0/37(LM_RL_Line04_pC0)  "<LM_RL_Line04_pC0>"
  Bus Selector2/37 -> TOS_ACC_P1/37(LM_RL_Line04_pC0)  "<LM_RL_Line04_pC0>"
  Bus Selector2/36 -> TOS_ACC_P1/36(LM_LR_Line04_pC0)  "<LM_LR_Line04_pC0>"
  Bus Selector2/35 -> TOS_ACC_P1/35(LM_LR_Line06_fCamValid)  "<LM_LR_Line06_fCamValid>"
  Bus Selector2/34 -> TOS_ACC_P1/34(LM_LR_Line05_fCamValid)  "<LM_LR_Line05_fCamValid>"
  Bus Selector2/33 -> TOS_ACC_P1/33(LM_LR_Line04_fCamValid)  "<LM_LR_Line04_fCamValid>"
  Bus Selector2/32 -> TOS_ACC_P1/32(LM_LR_Line06_pC2)  "<LM_LR_Line06_pC2>"
  Bus Selector2/31 -> TOS_ACC_P1/31(LM_LR_Line05_pC2)  "<LM_LR_Line05_pC2>"
  Bus Selector2/30 -> TOS_ACC_P1/30(LM_LR_Line04_pC2)  "<LM_LR_Line04_pC2>"
  Bus Selector2/29 -> TOS_ACC_P1/29(LM_LR_Line06_dDisEnd)  "<LM_LR_Line06_dDisEnd>"
  Bus Selector2/28 -> TOS_ACC_P1/28(LM_LR_Line06_dDisStart)  "<LM_LR_Line06_dDisStart>"
  Bus Selector2/27 -> TOS_ACC_P1/27(LM_LR_Line05_dDisEnd)  "<LM_LR_Line05_dDisEnd>"
  Bus Selector2/26 -> TOS_ACC_P1/26(LM_LR_Line05_dDisStart)  "<LM_LR_Line05_dDisStart>"
  Bus Selector2/25 -> TOS_ACC_P1/25(LM_LR_Line04_dDisEnd)  "<LM_LR_Line04_dDisEnd>"
  Bus Selector2/24 -> TOS_ACC_P1/24(LM_LR_Line04_dDisStart)  "<LM_LR_Line04_dDisStart>"
  Bus Selector2/23 -> TOS_ACC_P1/23(ACC_TargetP1_MovState_K2)  "<ACC_TargetP1_MovState_K2>"
  Bus Selector2/22 -> TOS_ACC_P1/22(ACC_TargetP1_MovState_K1)  "<ACC_TargetP1_MovState_K1>"
  Bus Selector2/21 -> TOS_ACC_P1/21(ACC_TargetP1_ID_K2)  "<ACC_TargetP1_ID_K2>"
  Bus Selector2/20 -> TOS_ACC_P1/20(ACC_TargetP1_ID_K1)  "<ACC_TargetP1_ID_K1>"
  Bus Selector2/19 -> TOS_ACC_P1/19(PIL_OverlapRatio)  "<PIL_OverlapRatio>"
  Bus Selector2/18 -> TOS_ACC_P1/18(SteerWheelAng)  "<SteerWheelAng>"
  Bus Selector2/17 -> TOS_ACC_P1/17(VIE_EgoVelocity)  "<VIE_EgoVelocity>"
  Bus Selector2/16 -> TOS_ACC_P1/16(Object_VY)  "<Object_VY>"
  Bus Selector2/15 -> TOS_ACC_P1/15(Object_VX)  "<Object_VX>"
  Bus Selector2/14 -> TOS_ACC_P1/14(PP_ObjFusType_FC_Confirm)  "<PP_ObjFusType_FC_Confirm>"
  Bus Selector2/13 -> TOS_ACC_P1/13(PP_ObjFusType_FR_Confirm)  "<PP_ObjFusType_FR_Confirm>"
  Bus Selector2/12 -> TOS_ACC_P1/12(PP_ObjFusType_FC_FR_Confirm)  "<PP_ObjFusType_FC_FR_Confirm>"
  Bus Selector2/1 -> TOS_ACC_P1/1(ACC_P0_P1_Index)  "<ACC_P0_P1_Index>"
  Bus Selector2/11 -> TOS_ACC_P1/11(Object_DY)  "<Object_DY>"
  Bus Selector2/6 -> TOS_ACC_P1/6(Object_HeadingAngle)  "<Object_HeadingAngle>"
  Bus Selector2/5 -> TOS_ACC_P1/5(PP_ObjMovingDirSignalProcessing)  "<PP_ObjMovingDirSignalProcessing>"
  Bus Selector2/10 -> TOS_ACC_P1/10(Object_ObstacleProb)  "<Object_ObstacleProb>"
  Bus Selector2/2 -> TOS_ACC_P1/2(Object_ID)  "<Object_ID>"
  Bus Selector2/9 -> TOS_ACC_P1/9(Object_Type)  "<Object_Type>"
  Bus Selector2/8 -> TOS_ACC_P1/8(TOS_TLJ_SameLaneConfirm_Flag)  "<TOS_TLJ_SameLaneConfirm_Flag>"
  Bus Selector2/7 -> TOS_ACC_P1/7(Object_DX)  "<Object_DX>"
  Bus Selector2/4 -> TOS_ACC_P1/4(object_MovingState)  "<Object_MovingState>"
  Bus Selector2/3 -> TOS_ACC_P1/3(Object_Fus_Type)  "<Object_Fus_Type>"
  TOS_ACC_P1/13(TOS_ACC_TrgMovDirFlag_6_ObserVale) -> Bus Creator2/12  "TOS_ACC_P1_TrgMovDirFlag_6_ObserVale"
  TOS_ACC_P1/17(TOS_ACC_DyConfirm_4_OverlapRatio_ObserVale) -> Bus Creator2/16  "TOS_ACC_P1_DyConfirm_4_OverlapRatio_ObserVale"
  TOS_ACC_P1/18(TOS_ACC_DyConfirm_5_OverlapConfirm_ObserVale) -> Bus Creator2/17  "TOS_ACC_P1_DyConfirm_5_OverlapConfirm_ObserVale"
  TOS_ACC_P1/19(TOS_ACC_DyConfirm_ALL_6_ObserVale) -> Bus Creator2/18  "TOS_ACC_P1_DyConfirm_ALL_6_ObserVale"
  LM_RL_Line04_pC1/1 -> Bus Creator/22  "LM_RL_Line04_pC1"
  LM_LR_Line04_pC1/1 -> Bus Creator/21  "LM_LR_Line04_pC1"
  Bus Selector/38 -> TOS_ACC_P0/38(LM_LR_Line04_pC1)  "<LM_LR_Line04_pC1>"
  Bus Selector/39 -> TOS_ACC_P0/39(LM_RL_Line04_pC1)  "<LM_RL_Line04_pC1>"

== system PubIfDecisionTOS_MDL/TOS_20201112/TOS_2012080320/TOS/ACC/TOS_ACCCurrentLane/ACC_Object_PreConfirm ==
  PP_ObjFusType_FC_FR_Confirm : Inport
  PP_ObjFusType_FR_Confirm : Inport  Port=2
  PP_ObjFusType_FC_Confirm : Inport  Port=3
  Object_ID : Inport  Port=4
  Obj_MovingState : Inport  Port=5
  Obj_Dx : Inport  Port=6
  Object_ObstacleProb : Inport  Port=7
  Object_DY : Inport  Port=8
  Object_Type : Inport  Port=9
  TOS_TLJ_SameLaneConfirm_Flag : Inport  Port=10
  LM_LR_Line04_fCamValid : Inport  Port=11
  LM_LR_Line05_fCamValid : Inport  Port=12
  LM_LR_Line06_fCamValid : Inport  Port=13
  PIL_OverlapRatio : Inport  Port=14
  LM_LR_Line04_dDisStart : Inport  Port=15
  LM_LR_Line04_dDisEnd : Inport  Port=16
  LM_LR_Line05_dDisStart : Inport  Port=17
  LM_LR_Line05_dDisEnd : Inport  Port=18
  LM_LR_Line06_dDisStart : Inport  Port=19
  LM_LR_Line06_dDisEnd : Inport  Port=20
  PP_REElementType : Inport  Port=21
  ACC_TargetP0_ID_K1 : Inport  Port=22
  ACC_TargetP0_Dx_K1 : Inport  Port=23
  ACC_P0_P1_Object_TargPreConfirm : Subsystem
  Bus Creator : BusCreator  Inputs=11
  Delay : Delay  InitialCondition=0
  Unit Delay : UnitDelay  SampleTime=-1  HasFrameUpgradeWarning=on
  Unit Delay1 : UnitDelay  InitialCondition=255  SampleTime=-1  HasFrameUpgradeWarning=on
  Unit Delay2 : UnitDelay  SampleTime=-1  HasFrameUpgradeWarning=on
  TOS_ACC_P0_P1_TargetPreConfirm : Outport
  wires:
  PP_ObjFusType_FR_Confirm/1 -> ACC_P0_P1_Object_TargPreConfirm/2(PP_ObjFusType_FR_Confirm)
  PP_ObjFusType_FC_FR_Confirm/1 -> ACC_P0_P1_Object_TargPreConfirm/1(PP_ObjFusType_FC_FR_Confirm)
  PP_ObjFusType_FC_Confirm/1 -> ACC_P0_P1_Object_TargPreConfirm/3(PP_ObjFusType_FC_Confirm)
  Object_ID/1 -> ACC_P0_P1_Object_TargPreConfirm/4(Object_ID)
  ACC_TargetP0_Dx_K1/1 -> Unit Delay1/1
  ACC_TargetP0_ID_K1/1 -> Unit Delay/1
  Object_DY/1 -> ACC_P0_P1_Object_TargPreConfirm/8(Object_DY)
  Object_ObstacleProb/1 -> ACC_P0_P1_Object_TargPreConfirm/7(Object_ObstacleProb)
  Obj_Dx/1 -> ACC_P0_P1_Object_TargPreConfirm/6(Obj_Dx)
  Obj_MovingState/1 -> ACC_P0_P1_Object_TargPreConfirm/5(Obj_MovingState)
  Object_Type/1 -> ACC_P0_P1_Object_TargPreConfirm/9(Object_ObjType)
  Bus Creator/1 -> TOS_ACC_P0_P1_TargetPreConfirm/1  "TOS_ACC_P0_P1_TargetPre_ObserVale"
  PIL_OverlapRatio/1 -> Delay/1, Unit Delay2/1, ACC_P0_P1_Object_TargPreConfirm/16(PIL_OverlapRatio)
  TOS_TLJ_SameLaneConfirm_Flag/1 -> ACC_P0_P1_Object_TargPreConfirm/10(TOS_TLJ_SameLaneConfirm_Flag)
  ACC_P0_P1_Object_TargPreConfirm/1(TOS_ACC_P0_P1_TargetPre_1_ConditionFlag_ObserVale) -> Bus Creator/1  "TOS_ACC_P0_P1_TargetPre_1_ConditionFlag_ObserVale"
  ACC_P0_P1_Object_TargPreConfirm/2(TOS_ACC_P0_P1_TargetPre_2_OverlapThre_ObserVale) -> Bus Creator/2  "TOS_ACC_P0_P1_TargetPre_2_OverlapThre_ObserVale"
  ACC_P0_P1_Object_TargPreConfirm/3(TOS_ACC_P0_P1_TargetPre_3_SameLane_Flag_ObserVale) -> Bus Creator/3  "TOS_ACC_P0_P1_TargetPre_3_SameLane_Flag_ObserVale"
  ACC_P0_P1_Object_TargPreConfirm/4(TOS_ACC_P0_P1_TargetPre_SameLaneFlag) -> Bus Creator/4  "TOS_ACC_P0_P1_TargetPre_SameLaneFlag"
  ACC_P0_P1_Object_TargPreConfirm/5(TOS_ACC_P0_P1_TargetPre_FiltFlag) -> Bus Creator/5  "TOS_ACC_P0_P1_TargetPreFiltFlag"
  ACC_P0_P1_Object_TargPreConfirm/6(TOS_ACC_P0_P1_TargetPre_FusionTypeFlag_ObserVale) -> Bus Creator/6  "TOS_ACC_P0_P1_TargetPre_FusionTypeFlag_ObserVale"
  ACC_P0_P1_Object_TargPreConfirm/7(TOS_ACC_P0_P1_TargetPre_PassedbyTarget_Flag_ObserVale) -> Bus Creator/7  "TOS_ACC_P0_P1_TargetPre_PassedbyTarget_Flag_ObserVale"
  ACC_P0_P1_Object_TargPreConfirm/8(TOS_ACC_P0_P1_TargetPre_FenceFlag_ObserVale) -> Bus Creator/8  "TOS_ACC_P0_P1_TargetPre_FenceFlag_ObserVale"
  ACC_P0_P1_Object_TargPreConfirm/9(TOS_ACC_P0_P1_TargetPre_ObjType_ObserVale) -> Bus Creator/9  "TOS_ACC_P0_P1_TargetPre_ObjType_ObserVale"
  ACC_P0_P1_Object_TargPreConfirm/10(TOS_ACC_P0_P1_TargetPre_OverlapThre_Val_ObserVale) -> Bus Creator/10  "TOS_ACC_P0_P1_TargetPre_OverlapThre_Val_ObserVale"
  Unit Delay/1 -> ACC_P0_P1_Object_TargPreConfirm/14(ACC_TargetP0_ID_K1)
  Unit Delay1/1 -> ACC_P0_P1_Object_TargPreConfirm/15(ACC_TargetP0_Dx_K1)
  Unit Delay2/1 -> ACC_P0_P1_Object_TargPreConfirm/17(PIL_OverlapRatio_K1)
  Delay/1 -> ACC_P0_P1_Object_TargPreConfirm/18(PIL_OverlapRatio_K2)
  LM_LR_Line04_fCamValid/1 -> ACC_P0_P1_Object_TargPreConfirm/11(LM_LR_Line04_fCamValid)
  LM_LR_Line05_fCamValid/1 -> ACC_P0_P1_Object_TargPreConfirm/12(LM_LR_Line05_fCamValid)
  LM_LR_Line06_fCamValid/1 -> ACC_P0_P1_Object_TargPreConfirm/13(LM_LR_Line06_fCamValid)
  LM_LR_Line06_dDisEnd/1 -> ACC_P0_P1_Object_TargPreConfirm/24(LM_LR_Line06_dDisEnd)
  LM_LR_Line04_dDisStart/1 -> ACC_P0_P1_Object_TargPreConfirm/19(LM_LR_Line04_dDisStart)
  LM_LR_Line04_dDisEnd/1 -> ACC_P0_P1_Object_TargPreConfirm/20(LM_LR_Line04_dDisEnd)
  LM_LR_Line05_dDisStart/1 -> ACC_P0_P1_Object_TargPreConfirm/21(LM_LR_Line05_dDisStart)
  LM_LR_Line05_dDisEnd/1 -> ACC_P0_P1_Object_TargPreConfirm/22(LM_LR_Line05_dDisEnd)
  LM_LR_Line06_dDisStart/1 -> ACC_P0_P1_Object_TargPreConfirm/23(LM_LR_Line06_dDisStart)
  PP_REElementType/1 -> ACC_P0_P1_Object_TargPreConfirm/25(PP_REElementType)
  ACC_P0_P1_Object_TargPreConfirm/11(TOS_ACC_P0_P1_TargetPre_REElementType_ObserVale) -> Bus Creator/11  "TOS_ACC_P0_P1_TargetPre_REElementType_ObserVale"

== system PubIfDecisionTOS_MDL/TOS_20201112/TOS_2012080320/TOS/ACC/TOS_ACCLeftLane/ACCTargetPO24Infor ==
  OFM_SignalVerification : Inport
  TOS_AddAttributes : Inport  Port=2
  TOS_ProbInLaneCalculat : Inport  Port=3
  TOS_ACCPO2TargetIndex : Inport  Port=4  OutDataTypeStr=uint8
  TOS_ACCPO4TargetIndex : Inport  Port=5  OutDataTypeStr=uint8
  Bus Creator : BusCreator  Inputs=3
  Bus Selector : BusSelector  OutputSignals=OFM_SignalVerification,TOS_AddAttributes,TOS_ProbInLaneCalculat
  Bus Selector1 : BusSelector  OutputSignals=OFM_SignalVerification,TOS_AddAttributes
  TOS_ACCPO2TargetInfor : Stateflow chart  TreatAsAtomicUnit=on
  TOS_ACCPO4TargetInfor : Stateflow chart  TreatAsAtomicUnit=on
  TOS_ACCPO2 : Outport  PortDimensions=1  BusOutputAsStruct=on
  TOS_ACCPO4 : Outport  Port=2
  wires:
  TOS_ACCPO2TargetIndex/1 -> TOS_ACCPO2TargetInfor/4(TOS_ACCPO2TargetIndex)
  Bus Selector/1 -> TOS_ACCPO2TargetInfor/1(OFM_SignalVerification)  "<OFM_SignalVerification>"
  Bus Selector/2 -> TOS_ACCPO2TargetInfor/2(TOS_AddAttributes)  "<TOS_AddAttributes>"
  TOS_AddAttributes/1 -> Bus Creator/2  "TOS_AddAttributes"
  OFM_SignalVerification/1 -> Bus Creator/1  "OFM_SignalVerification"
  Bus Creator/1 -> Bus Selector1/1, Bus Selector/1
  TOS_ProbInLaneCalculat/1 -> Bus Creator/3  "TOS_ProbInLaneCalculat"
  Bus Selector/3 -> TOS_ACCPO2TargetInfor/3(TOS_ProbInLaneCalculat)  "<TOS_ProbInLaneCalculat>"
  TOS_ACCPO2TargetInfor/1(TOS_ACCPO2TargetInfo) -> TOS_ACCPO2/1
  Bus Selector1/1 -> TOS_ACCPO4TargetInfor/1(OFM_SignalVerification)  "<OFM_SignalVerification>"
  Bus Selector1/2 -> TOS_ACCPO4TargetInfor/2(TOS_AddAttributes)  "<TOS_AddAttributes>"
  TOS_ACCPO4TargetIndex/1 -> TOS_ACCPO4TargetInfor/3(TOS_ACCPO4TargetIndex)
  TOS_ACCPO4TargetInfor/1(TOS_ACCPO4TargetInfo) -> TOS_ACCPO4/1

== system PubIfDecisionTOS_MDL/TOS_20201112/TOS_2012080320/TOS/ACC/TOS_ACCLeftLane/ACC_LeftLane_Target ==
  VIE_EgoVelocity : Inport
  OFM_SignalVerification : Inport  Port=2
  TOS_AddAttributes : Inport  Port=3
  TOS_ProbInLaneCalculat : Inport  Port=4
  TOS_VCAN_SignalVerification : Inport  Port=5
  TOS_ACC_P2_P4_Index : Inport  Port=6
  ACC_TargetP2_ID_K1 : Inport  Port=7
  ACC_TargetP2_MovState_K1 : Inport  Port=8
  ACC_TargetP4_ID_K1 : Inport  Port=9
  ACC_TargetP2_ID_K2 : InportShadow  Port=7
  ACC_TargetP2_MovState_K2 : InportShadow  Port=8
  ACC_TargetP4_ID_K2 : InportShadow  Port=9
  ACC_TargetP4_ID_K3 : InportShadow  Port=9
  Bus Creator : BusCreator  Inputs=14
  Bus Creator1 : BusCreator  Inputs=11
  Bus Creator2 : BusCreator  Inputs=11
  Bus Selector : BusSelector  OutputSignals=TOS_ACC_P2_P4_Index,OFM_SignalVerification.Object_ID,OFM_SignalVerification.Object_Fus_Type,OFM_SignalVerification.Object_MovingState,TOS_AddAttributes.PP_ObjMovingDirSignalProcessing,OFM_SignalVerification.Object_HeadingAngle,OFM_SignalVerification.Object_DX,OFM_SignalVerification.Object_Type,OFM_SignalVerification.Object_ObstacleProb,OFM_SignalVerification.Object_DY,TOS_AddAttributes.PP_ObjFusType_FC_FR_Confirm,TOS_AddAttributes.PP_ObjFusType_FR_Confirm,TOS_AddAttributes.PP_ObjFusType_FC_Confirm,OFM_SignalVerification.Object_VX,OFM_SignalVerification.Object_VY,VIE_EgoVelocity,TOS_VCAN_SignalVerification.SteerWheelAng,ACC_TargetP2_ID_K1,ACC_TargetP2_ID_K2,ACC_TargetP2_MovState_K1,ACC_TargetP2_MovState_K2
  Bus Selector1 : BusSelector  OutputSignals=TOS_ACC_P2_P4_Index,OFM_SignalVerification.Object_ID,OFM_SignalVerification.Object_Fus_Type,OFM_SignalVerification.Object_MovingState,TOS_AddAttributes.PP_ObjMovingDirSignalProcessing,OFM_SignalVerification.Object_HeadingAngle,OFM_SignalVerification.Object_DX,OFM_SignalVerification.Object_Type,OFM_SignalVerification.Object_ObstacleProb,OFM_SignalVerification.Object_DY,TOS_AddAttributes.PP_ObjFusType_FC_FR_Confirm,TOS_AddAttributes.PP_ObjFusType_FR_Confirm,TOS_AddAttributes.PP_ObjFusType_FC_Confirm,OFM_SignalVerification.Object_VX,OFM_SignalVerification.Object_VY,VIE_EgoVelocity,TOS_VCAN_SignalVerification.SteerWheelAng,ACC_TargetP4_ID_K1,ACC_TargetP4_ID_K2,ACC_TargetP4_MovState_K1,ACC_TargetP4_MovState_K2
  Bus Selector2 : BusSelector  OutputSignals=PP_MovingStateSignalProcessing
  Data Type Conversion{1..4} (4 alike) : DataTypeConversion  OutDataTypeStr=Enum: ObjectMovingState_E
  Delay{,3..4,7} (4 alike) : Delay  InitialCondition=0
  Delay{1..2,5..6} (4 alike) : Delay  DelayLength=1  InitialCondition=0
  Saturation : Saturate  UpperLimit=uint8(80)  LowerLimit=uint8(1)
  Selector1 : Selector  InputPortWidth=80  IndexOptions=Index vector (port)  Indices=[1 3]  OutputSizes=1
  Selector2 : Selector  InputPortWidth=80  IndexOptions=Index vector (port)  Indices=[1 3]  OutputSizes=1
  TOS_ACC_P2 : Subsystem
  TOS_ACC_P4 : Subsystem
  TOS_AddAttributes1 : InportShadow  Port=3
  Terminator : Terminator
  Terminator1 : Terminator
  TOS_ACC_P2_TragetIndex : Outport
  TOS_ACC_P4_TragetIndex : Outport  Port=2
  wires:
  TOS_AddAttributes/1 -> Bus Creator/3  "TOS_AddAttributes"
  OFM_SignalVerification/1 -> Bus Creator/2
  VIE_EgoVelocity/1 -> Bus Creator/1  "VIE_EgoVelocity"
  TOS_ProbInLaneCalculat/1 -> Bus Creator/4  "TOS_ProbInLaneCalculat"
  TOS_ACC_P2/1(TOS_ACC_P2_Index) -> TOS_ACC_P2_TragetIndex/1  "TOS_ACC_P2_TragetIndex"
  Bus Creator1/1 -> Terminator/1  "TOS_ACC_P2_ObserVale"
  TOS_ACC_P2_P4_Index/1 -> Bus Creator/6  "TOS_ACC_P2_P4_Index"
  TOS_VCAN_SignalVerification/1 -> Bus Creator/5  "TOS_VCAN_SignalVerification"
  Delay1/1 -> Bus Creator/7  "ACC_TargetP2_ID_K1"
  Delay/1 -> Bus Creator/8  "ACC_TargetP2_ID_K2"
  Delay2/1 -> Data Type Conversion2/1
  Data Type Conversion1/1 -> Bus Creator/10  "ACC_TargetP2_MovState_K2"
  ACC_TargetP2_MovState_K2/1 -> Delay3/1
  Data Type Conversion2/1 -> Bus Creator/9  "ACC_TargetP2_MovState_K1"
  Delay3/1 -> Data Type Conversion1/1
  ACC_TargetP2_ID_K2/1 -> Delay/1
  ACC_TargetP2_ID_K1/1 -> Delay1/1
  ACC_TargetP2_MovState_K1/1 -> Delay2/1
  Bus Selector/1 -> TOS_ACC_P2/1(TOS_ACC_P2_P4_Index)  "<TOS_ACC_P2_P4_Index>"
  Bus Selector/2 -> TOS_ACC_P2/2(Object_ID)  "<Object_ID>"
  Bus Selector/3 -> TOS_ACC_P2/3(Object_Fus_Type)  "<Object_Fus_Type>"
  Bus Selector/4 -> TOS_ACC_P2/4(object_MovingState)  "<Object_MovingState>"
  Bus Selector/5 -> TOS_ACC_P2/5(PP_ObjMovingDirSignalProcessing)  "<PP_ObjMovingDirSignalProcessing>"
  Bus Selector/6 -> TOS_ACC_P2/6(Object_HeadingAngle)  "<Object_HeadingAngle>"
  Bus Selector/7 -> TOS_ACC_P2/7(Object_DX)  "<Object_DX>"
  Bus Selector/8 -> TOS_ACC_P2/8(Object_Type)  "<Object_Type>"
  Bus Selector/9 -> TOS_ACC_P2/9(Object_ObstacleProb)  "<Object_ObstacleProb>"
  Bus Selector/10 -> TOS_ACC_P2/10(Object_DY)  "<Object_DY>"
  Bus Selector/11 -> TOS_ACC_P2/11(PP_ObjFusType_FC_FR_Confirm)  "<PP_ObjFusType_FC_FR_Confirm>"
  Bus Selector/12 -> TOS_ACC_P2/12(PP_ObjFusType_FR_Confirm)  "<PP_ObjFusType_FR_Confirm>"
  Bus Selector/13 -> TOS_ACC_P2/13(PP_ObjFusType_FC_Confirm)  "<PP_ObjFusType_FC_Confirm>"
  Bus Selector/14 -> TOS_ACC_P2/14(Object_VX)  "<Object_VX>"
  Bus Selector/15 -> TOS_ACC_P2/15(Object_VY)  "<Object_VY>"
  Bus Selector/16 -> TOS_ACC_P2/16(VIE_EgoVelocity)  "<VIE_EgoVelocity>"
  Bus Selector/17 -> TOS_ACC_P2/17(SteerWheelAng)  "<SteerWheelAng>"
  Bus Selector/18 -> TOS_ACC_P2/18(ACC_TargetP2_ID_K1)  "<ACC_TargetP2_ID_K1>"
  Bus Selector/19 -> TOS_ACC_P2/19(ACC_TargetP2_ID_K2)  "<ACC_TargetP2_ID_K2>"
  Bus Selector/20 -> TOS_ACC_P2/20(ACC_TargetP2_MovState_K1)  "<ACC_TargetP2_MovState_K1>"
  Bus Selector/21 -> TOS_ACC_P2/21(ACC_TargetP2_MovState_K2)  "<ACC_TargetP2_MovState_K2>"
  TOS_ACC_P2/5(TOS_ACC_ObjType_ObserVale) -> Bus Creator1/4  "TOS_ACC_P2_ObjType_ObserVale"
  TOS_ACC_P2/4(TOS_ACC_TargetDxConfirm_ObserVale) -> Bus Creator1/3  "TOS_ACC_P2_TargetDxConfirm_ObserVale"
  TOS_ACC_P2/6(TOS_ACC_ObstacleProb_ObserVale) -> Bus Creator1/5  "TOS_ACC_P2_ObstacleProb_ObserVale"
  TOS_ACC_P2/3(TOS_ACC_TrgMovDir_ObserVale) -> Bus Creator1/2  "TOS_ACC_P2_TrgMovDir_ObserVale"
  TOS_ACC_P2/7(TOS_ACC_TrgMovDirFlag_1_ObserVale) -> Bus Creator1/6  "TOS_ACC_P2_TrgMovDirFlag_1_ObserVale"
  TOS_ACC_P2/2(TOS_ACC_FusionType_ObserVale) -> Bus Creator1/1  "TOS_ACC_P2_FusionType_ObserVale"
  TOS_ACC_P2/8(TOS_ACC_TrgMovDirFlag_2_ObserVale) -> Bus Creator1/7  "TOS_ACC_P2_TrgMovDirFlag_2_ObserVale"
  TOS_ACC_P2/9(TOS_ACC_TrgMovDirFlag_3_ObserVale) -> Bus Creator1/8  "TOS_ACC_P2_TrgMovDirFlag_3_ObserVale"
  TOS_ACC_P2/10(TOS_ACC_TrgMovDirFlag_4_ObserVale) -> Bus Creator1/9  "TOS_ACC_P2_TrgMovDirFlag_4_ObserVale"
  TOS_ACC_P2/11(TOS_ACC_TrgMovDirFlag_5_ObserVale) -> Bus Creator1/10  "TOS_ACC_P2_TrgMovDirFlag_5_ObserVale"
  TOS_ACC_P2/12(TOS_ACC_TrgMovDirFlag_6_ObserVale) -> Bus Creator1/11  "TOS_ACC_P2_TrgMovDirFlag_6_ObserVale"
  Selector1/1 -> Delay6/1
  ACC_TargetP4_ID_K1/1 -> Delay5/1
  ACC_TargetP4_ID_K2/1 -> Delay4/1
  Delay7/1 -> Data Type Conversion4/1
  Data Type Conversion3/1 -> Bus Creator/13  "ACC_TargetP4_MovState_K1"
  Selector2/1 -> Delay7/1
  Data Type Conversion4/1 -> Bus Creator/14  "ACC_TargetP4_MovState_K2"
  Delay6/1 -> Data Type Conversion3/1
  Delay4/1 -> Bus Creator/12  "ACC_TargetP4_ID_K2"
  Delay5/1 -> Bus Creator/11  "ACC_TargetP4_ID_K1"
  Bus Creator/1 -> Bus Selector1/1, Bus Selector/1
  TOS_ACC_P4/12(TOS_ACC_TrgMovDirFlag_6_ObserVale) -> Bus Creator2/11  "TOS_ACC_P4_TrgMovDirFlag_6_ObserVale"
  TOS_ACC_P4/11(TOS_ACC_TrgMovDirFlag_5_ObserVale) -> Bus Creator2/10  "TOS_ACC_P4_TrgMovDirFlag_5_ObserVale"
  TOS_ACC_P4/10(TOS_ACC_TrgMovDirFlag_4_ObserVale) -> Bus Creator2/9  "TOS_ACC_P4_TrgMovDirFlag_4_ObserVale"
  TOS_ACC_P4/9(TOS_ACC_TrgMovDirFlag_3_ObserVale) -> Bus Creator2/8  "TOS_ACC_P4_TrgMovDirFlag_3_ObserVale"
  TOS_ACC_P4/8(TOS_ACC_TrgMovDirFlag_2_ObserVale) -> Bus Creator2/7  "TOS_ACC_P4_TrgMovDirFlag_2_ObserVale"
  TOS_ACC_P4/2(TOS_ACC_FusionType_ObserVale) -> Bus Creator2/1  "TOS_ACC_P4_FusionType_ObserVale"
  TOS_ACC_P4/7(TOS_ACC_TrgMovDirFlag_1_ObserVale) -> Bus Creator2/6  "TOS_ACC_P4_TrgMovDirFlag_1_ObserVale"
  TOS_ACC_P4/3(TOS_ACC_TrgMovDir_ObserVale) -> Bus Creator2/2  "TOS_ACC_P4_TrgMovDir_ObserVale"
  TOS_ACC_P4/6(TOS_ACC_ObstacleProb_ObserVale) -> Bus Creator2/5  "TOS_ACC_P4_ObstacleProb_ObserVale"
  TOS_ACC_P4/4(TOS_ACC_TargetDxConfirm_ObserVale) -> Bus Creator2/3  "TOS_ACC_P4_TargetDxConfirm_ObserVale"
  TOS_ACC_P4/5(TOS_ACC_ObjType_ObserVale) -> Bus Creator2/4  "TOS_ACC_P4_ObjType_ObserVale"
  Bus Selector1/21 -> TOS_ACC_P4/21(ACC_TargetP4_MovState_K2)  "<ACC_TargetP4_MovState_K2>"
  Bus Selector1/20 -> TOS_ACC_P4/20(ACC_TargetP4_MovState_K1)  "<ACC_TargetP4_MovState_K1>"
  Bus Selector1/19 -> TOS_ACC_P4/19(ACC_TargetP4_ID_K2)  "<ACC_TargetP4_ID_K2>"
  Bus Selector1/18 -> TOS_ACC_P4/18(ACC_TargetP4_ID_K1)  "<ACC_TargetP4_ID_K1>"
  Bus Selector1/17 -> TOS_ACC_P4/17(SteerWheelAng)  "<SteerWheelAng>"
  Bus Selector1/16 -> TOS_ACC_P4/16(VIE_EgoVelocity)  "<VIE_EgoVelocity>"
  Bus Selector1/15 -> TOS_ACC_P4/15(Object_VY)  "<Object_VY>"
  Bus Selector1/14 -> TOS_ACC_P4/14(Object_VX)  "<Object_VX>"
  Bus Selector1/13 -> TOS_ACC_P4/13(PP_ObjFusType_FC_Confirm)  "<PP_ObjFusType_FC_Confirm>"
  Bus Selector1/12 -> TOS_ACC_P4/12(PP_ObjFusType_FR_Confirm)  "<PP_ObjFusType_FR_Confirm>"
  Bus Selector1/11 -> TOS_ACC_P4/11(PP_ObjFusType_FC_FR_Confirm)  "<PP_ObjFusType_FC_FR_Confirm>"
  Bus Selector1/10 -> TOS_ACC_P4/10(Object_DY)  "<Object_DY>"
  Bus Selector1/9 -> TOS_ACC_P4/9(Object_ObstacleProb)  "<Object_ObstacleProb>"
  Bus Selector1/8 -> TOS_ACC_P4/8(Object_Type)  "<Object_Type>"
  Bus Selector1/7 -> TOS_ACC_P4/7(Object_DX)  "<Object_DX>"
  Bus Selector1/6 -> TOS_ACC_P4/6(Object_HeadingAngle)  "<Object_HeadingAngle>"
  Bus Selector1/5 -> TOS_ACC_P4/5(PP_ObjMovingDirSignalProcessing)  "<PP_ObjMovingDirSignalProcessing>"
  Bus Selector1/4 -> TOS_ACC_P4/4(object_MovingState)  "<Object_MovingState>"
  Bus Selector1/3 -> TOS_ACC_P4/3(Object_Fus_Type)  "<Object_Fus_Type>"
  Bus Selector1/2 -> TOS_ACC_P4/2(Object_ID)  "<Object_ID>"
  Bus Selector1/1 -> TOS_ACC_P4/1(TOS_ACC_P2_P4_Index)  "<TOS_ACC_P2_P4_Index>"
  Bus Creator2/1 -> Terminator1/1  "TOS_ACC_P4_ObserVale"
  TOS_ACC_P4/1(TOS_ACC_P4_Index) -> TOS_ACC_P4_TragetIndex/1  "TOS_ACC_P4_TragetIndex"
  TOS_AddAttributes1/1 -> Bus Selector2/1  "TOS_AddAttributes"
  Bus Selector2/1 -> Selector1/1, Selector2/1  "<PP_MovingStateSignalProcessing>"
  ACC_TargetP4_ID_K3/1 -> Saturation/1
  Saturation/1 -> Selector1/2, Selector2/2
